simulink model "Simulink3"  (Simulink 5.0)
settings: Solver=ode45  StartTime=0.0  StopTime=50.0  RelTol=1e-5
libraries: simulink x1
settings Model: LastModifiedBy=stevel

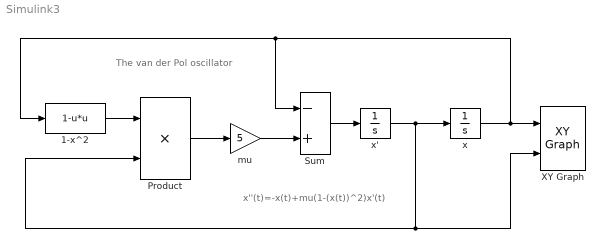
== system Simulink3 ==
  note: x''(t)=-x(t)+mu(1-(x(t))^2)x'(t)
  note: The van der Pol oscillator
  1-x^2 : Fcn  Expr=1-u*u
  Product : Product  SaturateOnIntegerOverflow=on
  Sum : Sum  Inputs=-+  SaturateOnIntegerOverflow=on
  XY Graph : simulink/Sinks/XY Graph  xmin=-3  xmax=3  ymin=-10  ymax=10  st=-1
  mu : Gain  Gain=5  SaturateOnIntegerOverflow=on
  x : Integrator  InitialCondition=2
  x' : Integrator
  wires:
  mu/1 -> Sum/2
  Sum/1 -> x'/1
  x'/1 -> x/1, Product/2, XY Graph/2
  x/1 -> Sum/1, 1-x^2/1, XY Graph/1
  Product/1 -> mu/1
  1-x^2/1 -> Product/1
